simulink model "thermal"  (R2016b)
settings: Solver=VariableStepAuto  StartTime=0.0  StopTime=10.0  RelTol=1e-3
libraries: simulink x1
settings Model: Creator=charAn  LastModifiedBy=charAn

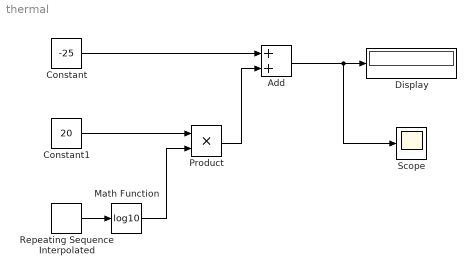
== system thermal ==
  Add : Sum
  Constant : Constant  Value=-25
  Constant1 : Constant  Value=20
  Display : Display
  Math Function : Math  Operator=log10  SaturateOnIntegerOverflow=on
  Product : Product
  Repeating Sequence Interpolated : simulink/Sources/Repeating Sequence Interpolated  OutValues=[0 200 10200 20200 30200 40200 50200 60200 70200 80200 90200 100200 110200 120200 130200 140200 150200 160200 170200 180200 190200 200200]  TimeValues=[0 10 20 30 40 50 60 70 80 90 100 120 140 160 180 200 220 240 260 280 300 320 ]  LookUpMeth=Interpolation-Use End Values  tsamp=0.01  OutMin=[]  OutMax=[]  OutDataTypeStr=double  OutputDataTypeScalingMode=double  OutDataType=fixdt(0,8)  OutScaling=2^-10
  Scope : Scope
  wires:
  Constant/1 -> Add/1
  Repeating Sequence Interpolated/1 -> Math Function/1
  Math Function/1 -> Product/2
  Constant1/1 -> Product/1
  Product/1 -> Add/2
  Add/1 -> Scope/1, Display/1
